simulink model "Zamora22210432P2"  (R2023a)
settings: Solver=ode15s  StartTime=0.0  StopTime=30  MaxStep=1E-3  RelTol=1e-3
libraries: slpidlib x1
settings Model: NumberOfSteps=15  Creator=Michelle  LastModifiedBy=Michelle
settings DataIOCC: ReturnWorkspaceOutputs=off  TimeSaveName=t
settings DebuggingCC: AlgebraicLoopMsg=none  ArtificialAlgebraicLoopMsg=none  MaxConsecutiveZCsMsg=none  ModelReferenceExtraNoncontSigs=none  OperatingPointInterfaceChecksumMismatchMsg=none

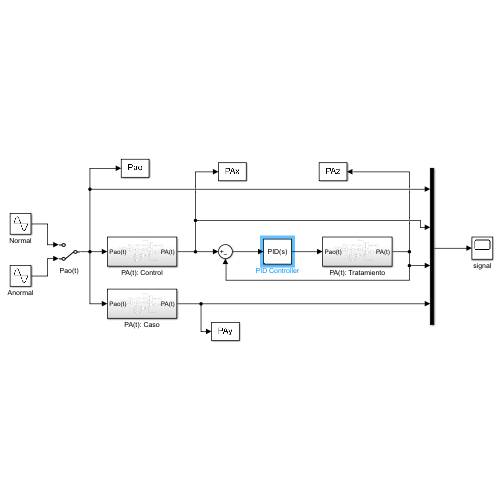
[thumbnail: Simulink's stored preview of the top-level diagram]
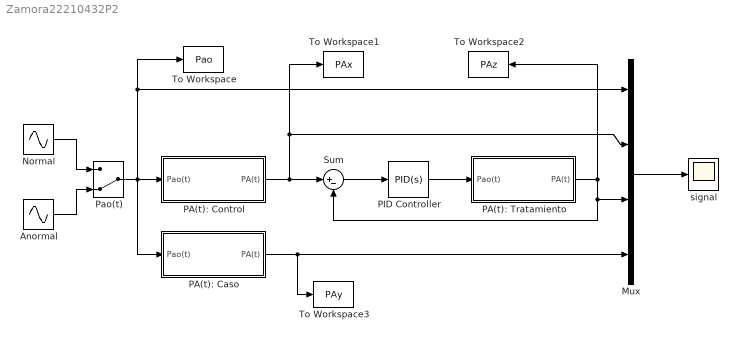
== system Zamora22210432P2 ==
  Anormal : Sin  Amplitude=1.5  Frequency=pi  SampleTime=0
  Mux : Mux
  Normal : Sin  Amplitude=2.5  Frequency=pi/2  SampleTime=0
  PA(t): Caso : Subsystem
  PA(t): Control : Subsystem
  PA(t): Tratamiento : Subsystem
  PID Controller : slpidlib/PID Controller  Controller=PID  Form=Parallel  TimeDomain=Continuous-time  UseExternalTs=off  SampleTime=-1  IntegratorMethod=Forward Euler  FilterMethod=Forward Euler  ControllerParametersSource=internal  P=177.954  I=4222.043  UseKiTs=off  D=0.951  N=17997.2909612851  UseFilter=on  TunerSelectOption=Transfer Function Based (PID Tuner App)  InitialConditionSource=internal  InitialConditionForIntegrator=0  InitialConditionForFilter=0  DifferentiatorICPrevScaledInput=0  ExternalReset=none  TrackingMode=off  Kt=1  LimitOutput=off  SatLimitsSource=internal  UpperSaturationLimit=inf  LowerSaturationLimit=-inf  LinearizeAsGain=on  AntiWindupMode=none  Kb=1  LimitIntegrator=off  UpperIntegratorSaturationLimit=inf  LowerIntegratorSaturationLimit=-inf  POutMin=[]  POutMax=[]  IOutMin=[]  IOutMax=[]  DOutMin=[]  DOutMax=[]  NOutMin=[]  NOutMax=[]  SumOutMin=[]  SumOutMax=[]  SaturationOutMin=[]  SaturationOutMax=[]  PParamMin=[]  PParamMax=[]  IParamMin=[]  IParamMax=[]  DParamMin=[]  DParamMax=[]  NParamMin=[]  NParamMax=[]  KbParamMin=[]  KbParamMax=[]  KtParamMin=[]  KtParamMax=[]  KbOutMin=[]  KbOutMax=[]  KtOutMin=[]  KtOutMax=[]  IntegratorOutMin=[]  IntegratorOutMax=[]  FilterOutMin=[]  FilterOutMax=[]  SumI1OutMin=[]  SumI1OutMax=[]  SumI2OutMin=[]  SumI2OutMax=[]  SumI3OutMin=[]  SumI3OutMax=[]  SumI4OutMin=[]  SumI4OutMax=[]  SumDOutMin=[]  SumDOutMax=[]  DifferentiatorOutMin=[]  DifferentiatorOutMax=[]  FilterDiffOutCoefMin=[]  FilterDiffOutCoefMax=[]  ReciprocalOutMin=[]  ReciprocalOutMax=[]  SumDenOutMin=[]  SumDenOutMax=[]  SumNumOutMin=[]  SumNumOutMax=[]  DivideOutMin=[]  DivideOutMax=[]  UdiffTsProdOutMin=[]  UdiffTsProdOutMax=[]  NTsProdOutMin=[]  NTsProdOutMax=[]  UintegralTsProdOutMin=[]  UintegralTsProdOutMax=[]  UngainTsProdOutMin=[]  UngainTsProdOutMax=[]  ClampingZeroOutDataTypeStr=Inherit: Inherit via back propagation  ClampingZeroOutMin=[]  ClampingZeroOutMax=[]  FilterDenConstantOutDataTypeStr=Inherit: Inherit via back propagation  FilterDenConstantOutMin=[]  FilterDenConstantOutMax=[]  PCopyOutDataTypeStr=Inherit: Inherit via back propagation  PCopyOutMin=[]  PCopyOutMax=[]  NCopyOutDataTypeStr=Inherit: Inherit via back propagation  NCopyOutMin=[]  NCopyOutMax=[]  IntegratorContinuousStateAttributes=''  IntegratorStateMustResolveToSignalObject=off  IntegratorRTWStateStorageClass=Auto  FilterContinuousStateAttributes=''  FilterStateMustResolveToSignalObject=off  FilterRTWStateStorageClass=Auto  ParallelPVariant=InternalParameters  IdealPVariant=Disabled  IVariant=InternalParameters  DVariant=InternalParameters  IntegratorVariant=Continuous  SatVariant=Disabled  AWVariant=Passthrough  PCopyVariant=Disabled  TRVariant=Disabled  FdbkBlocksVariant=Forward  IdealPFdbkVariant=Disabled  SatFdbkVariant=Disabled  DerivativeFilterVariant=ContFilter  NVariant=InternalParameters  NCopyVariant=Disabled  FilterICVariant=InternalICsFilter  IntegratorICVariant=InternalICs  ExternalResetVariant=Disabled  TRSumVariant=Passthrough  SumFdbkVariant=Disabled  SumVariant=Sum_PID  TsampFilterVariant=InternalTs  TsampNgainVariant=Passthrough  TsampIntegralVariant=Disabled_SignalSpec  ExternalSaturationOutDataTypeStr=Inherit: Same as second input
  Pao(t) : ManualSwitch  CurrentSetting=0
  Sum : Sum  Inputs=|+-
  To Workspace : ToWorkspace  VariableName=Pao  SampleTime=-1
  To Workspace1 : ToWorkspace  VariableName=PAx  SampleTime=-1
  To Workspace2 : ToWorkspace  VariableName=PAz  SampleTime=-1
  To Workspace3 : ToWorkspace  VariableName=PAy  SampleTime=-1
  signal : Scope
  wires:
  Mux/1 -> signal/1
  PID Controller/1 -> PA(t): Tratamiento/1(Pao(t))
  PA(t): Control/1(PA(t)) -> Sum/1, To Workspace1/1, Mux/2
  Sum/1 -> PID Controller/1
  PA(t): Caso/1(PA(t)) -> To Workspace3/1, Mux/4
  Normal/1 -> Pao(t)/1
  Anormal/1 -> Pao(t)/2
  Pao(t)/1 -> Mux/1, To Workspace/1, PA(t): Control/1(Pao(t)), PA(t): Caso/1(Pao(t))
  PA(t): Tratamiento/1(PA(t)) -> To Workspace2/1, Mux/3, Sum/2

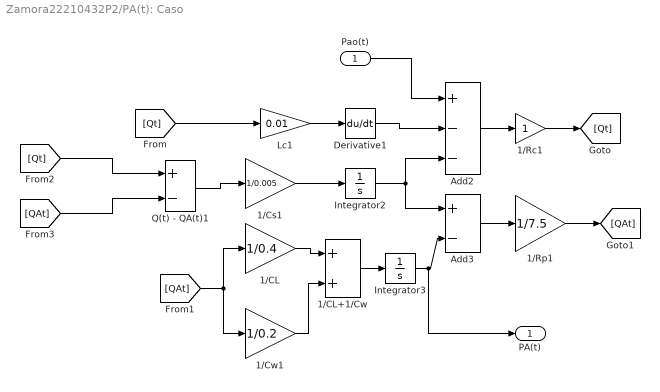
== system Zamora22210432P2/PA(t): Caso ==
  Pao(t) : Inport
  1/CL : Gain  Gain=1/0.4
  1/CL+1/Cw : Sum
  1/Cs1 : Gain  Gain=1/0.005
  1/Cw1 : Gain  Gain=1/0.2
  1/Rc1 : Gain
  1/Rp1 : Gain  Gain=1/7.5
  Add2 : Sum  Inputs=+--
  Add3 : Sum  Inputs=+-
  Derivative1 : Derivative
  Integrator2 : Integrator
  Integrator3 : Integrator
  Lc1 : Gain  Gain=0.01
  Q(t) - QA(t)1 : Sum  Inputs=+-
  PA(t) : Outport
  wires:
  1/Rc1/1 -> [Qt]
  [QAt] -> Q(t) - QA(t)1/2
  [QAt] -> 1/Cw1/1, 1/CL/1
  1/Cs1/1 -> Integrator2/1
  Integrator3/1 -> PA(t)/1, Add3/2
  Add3/1 -> 1/Rp1/1
  Integrator2/1 -> Add3/1, Add2/3
  1/CL/1 -> 1/CL+1/Cw/1
  Q(t) - QA(t)1/1 -> 1/Cs1/1
  1/CL+1/Cw/1 -> Integrator3/1
  Add2/1 -> 1/Rc1/1
  Lc1/1 -> Derivative1/1
  Derivative1/1 -> Add2/2
  Pao(t)/1 -> Add2/1
  1/Cw1/1 -> 1/CL+1/Cw/2
  [Qt] -> Q(t) - QA(t)1/1
  [Qt] -> Lc1/1
  1/Rp1/1 -> [QAt]

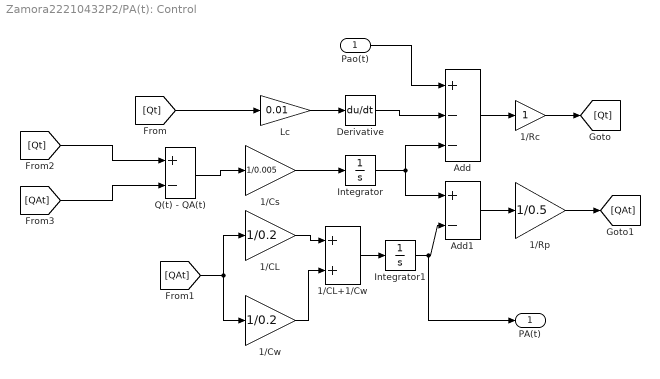
== system Zamora22210432P2/PA(t): Control ==
  Pao(t) : Inport
  1/CL : Gain  Gain=1/0.2
  1/CL+1/Cw : Sum
  1/Cs : Gain  Gain=1/0.005
  1/Cw : Gain  Gain=1/0.2
  1/Rc : Gain
  1/Rp : Gain  Gain=1/0.5
  Add : Sum  Inputs=+--
  Add1 : Sum  Inputs=+-
  Derivative : Derivative
  Integrator : Integrator
  Integrator1 : Integrator
  Lc : Gain  Gain=0.01
  Q(t) - QA(t) : Sum  Inputs=+-
  PA(t) : Outport
  wires:
  Lc/1 -> Derivative/1
  Add/1 -> 1/Rc/1
  Pao(t)/1 -> Add/1
  Q(t) - QA(t)/1 -> 1/Cs/1
  Derivative/1 -> Add/2
  1/Cw/1 -> 1/CL+1/Cw/2
  Integrator/1 -> Add1/1, Add/3
  1/Cs/1 -> Integrator/1
  Integrator1/1 -> PA(t)/1, Add1/2
  Add1/1 -> 1/Rp/1
  1/CL/1 -> 1/CL+1/Cw/1
  1/CL+1/Cw/1 -> Integrator1/1
  [Qt] -> Lc/1
  1/Rc/1 -> [Qt]
  1/Rp/1 -> [QAt]
  [QAt] -> 1/Cw/1, 1/CL/1
  [Qt] -> Q(t) - QA(t)/1
  [QAt] -> Q(t) - QA(t)/2

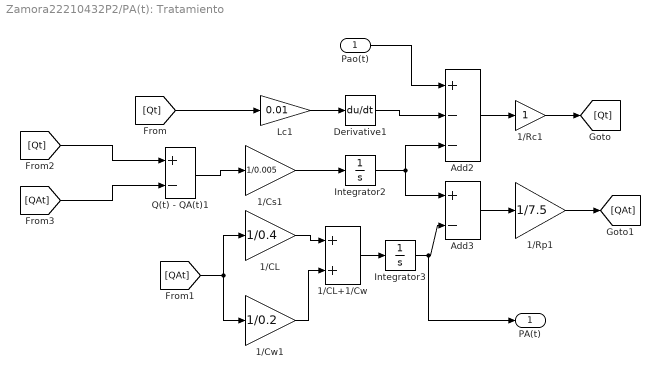
== system Zamora22210432P2/PA(t): Tratamiento ==
  Pao(t) : Inport
  1/CL : Gain  Gain=1/0.4
  1/CL+1/Cw : Sum
  1/Cs1 : Gain  Gain=1/0.005
  1/Cw1 : Gain  Gain=1/0.2
  1/Rc1 : Gain
  1/Rp1 : Gain  Gain=1/7.5
  Add2 : Sum  Inputs=+--
  Add3 : Sum  Inputs=+-
  Derivative1 : Derivative
  Integrator2 : Integrator
  Integrator3 : Integrator
  Lc1 : Gain  Gain=0.01
  Q(t) - QA(t)1 : Sum  Inputs=+-
  PA(t) : Outport
  wires:
  1/Rc1/1 -> [Qt]
  [QAt] -> Q(t) - QA(t)1/2
  [QAt] -> 1/Cw1/1, 1/CL/1
  1/Cs1/1 -> Integrator2/1
  Integrator3/1 -> PA(t)/1, Add3/2
  Add3/1 -> 1/Rp1/1
  Integrator2/1 -> Add3/1, Add2/3
  1/CL/1 -> 1/CL+1/Cw/1
  Q(t) - QA(t)1/1 -> 1/Cs1/1
  1/CL+1/Cw/1 -> Integrator3/1
  Add2/1 -> 1/Rc1/1
  Lc1/1 -> Derivative1/1
  Derivative1/1 -> Add2/2
  Pao(t)/1 -> Add2/1
  1/Cw1/1 -> 1/CL+1/Cw/2
  [Qt] -> Q(t) - QA(t)1/1
  [Qt] -> Lc1/1
  1/Rp1/1 -> [QAt]
